simulink model "WSCC_1SM_1GFM_1GFL"  (R2020b)
settings: Solver=VariableStepAuto  StartTime=0.0  StopTime=simlt.T_stop  RelTol=1e-3
undefined symbols (not defined in the file or in its folder): simlt
libraries: powerlib x45, G2ELib_V1 x3, eePowerMeasurement x3
settings Model: Creator=keladaf  LastModifiedBy=keladaf
settings DataIOCC: ReturnWorkspaceOutputs=off
settings DebuggingCC: UnconnectedInputMsg=none  UnconnectedOutputMsg=none  UnconnectedLineMsg=none

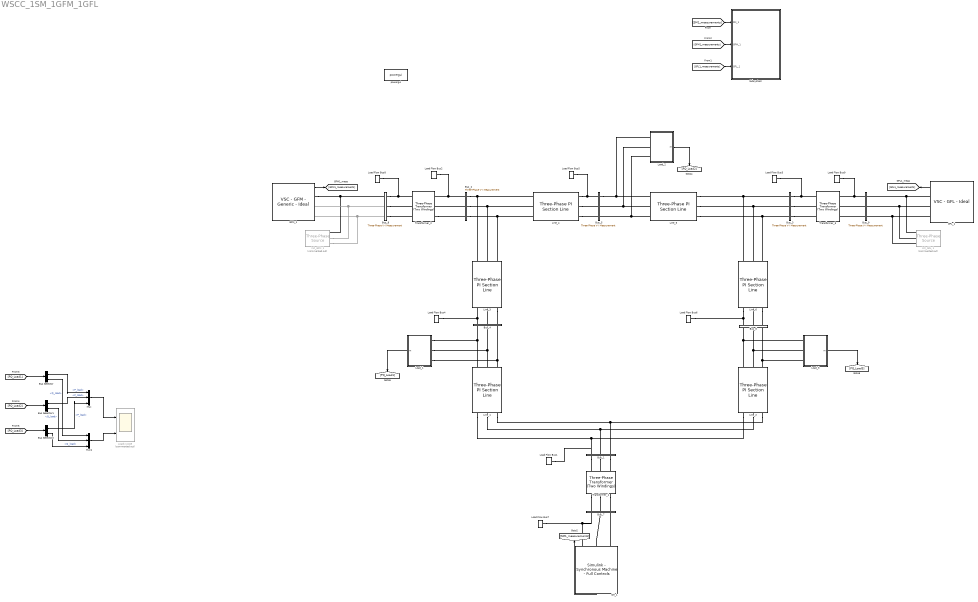
== system WSCC_1SM_1GFM_1GFL ==
  Bus Selector : BusSelector  OutputSignals=P_load,Q_load
  Bus Selector1 : BusSelector  OutputSignals=P_load,Q_load
  Bus Selector2 : BusSelector  OutputSignals=P_load,Q_load
  Bus_1 : powerlib/Measurements/Three-Phase V-I Measurement  VoltageMeasurement=phase-to-ground  SetLabelV=on  LabelV=V_Bus1  Vpu=off  VpuLL=off  CurrentMeasurement=yes  SetLabelI=on  LabelI=I_Bus1  Ipu=off  Pbase=100e6  Vbase=500e3  OutputType=Complex  PhasorSimulation=off  PSBequivalent=0
  Bus_2 : powerlib/Measurements/Three-Phase V-I Measurement  VoltageMeasurement=phase-to-ground  SetLabelV=on  LabelV=V_Bus2  Vpu=off  VpuLL=off  CurrentMeasurement=yes  SetLabelI=on  LabelI=I_Bus2  Ipu=off  Pbase=100e6  Vbase=500e3  OutputType=Complex  PhasorSimulation=off  PSBequivalent=0
  Bus_3 : powerlib/Measurements/Three-Phase V-I Measurement  VoltageMeasurement=phase-to-ground  SetLabelV=on  LabelV=V_Bus3  Vpu=off  VpuLL=off  CurrentMeasurement=yes  SetLabelI=on  LabelI=I_Bus3  Ipu=off  Pbase=100e6  Vbase=500e3  OutputType=Complex  PhasorSimulation=off  PSBequivalent=0
  Bus_4 : powerlib/Measurements/Three-Phase V-I Measurement  VoltageMeasurement=phase-to-ground  SetLabelV=on  LabelV=V_Bus4  Vpu=off  VpuLL=off  CurrentMeasurement=yes  SetLabelI=on  LabelI=I_Bus4  Ipu=off  Pbase=100e6  Vbase=500e3  OutputType=Complex  PhasorSimulation=off  PSBequivalent=0
  Bus_5 : powerlib/Measurements/Three-Phase V-I Measurement  VoltageMeasurement=phase-to-ground  SetLabelV=on  LabelV=V_Bus5  Vpu=off  VpuLL=off  CurrentMeasurement=yes  SetLabelI=on  LabelI=I_Bus5  Ipu=off  Pbase=100e6  Vbase=500e3  OutputType=Complex  PhasorSimulation=off  PSBequivalent=0
  Bus_6 : powerlib/Measurements/Three-Phase V-I Measurement  VoltageMeasurement=phase-to-ground  SetLabelV=on  LabelV=V_Bus6  Vpu=off  VpuLL=off  CurrentMeasurement=yes  SetLabelI=on  LabelI=I_Bus6  Ipu=off  Pbase=100e6  Vbase=500e3  OutputType=Complex  PhasorSimulation=off  PSBequivalent=0
  Bus_7 : powerlib/Measurements/Three-Phase V-I Measurement  VoltageMeasurement=phase-to-ground  SetLabelV=on  LabelV=V_Bus7  Vpu=off  VpuLL=off  CurrentMeasurement=yes  SetLabelI=on  LabelI=I_Bus7  Ipu=off  Pbase=100e6  Vbase=500e3  OutputType=Complex  PhasorSimulation=off  PSBequivalent=0
  Bus_8 : powerlib/Measurements/Three-Phase V-I Measurement  VoltageMeasurement=phase-to-ground  SetLabelV=on  LabelV=V_Bus8  Vpu=off  VpuLL=off  CurrentMeasurement=yes  SetLabelI=on  LabelI=I_Bus8  Ipu=off  Pbase=100e6  Vbase=500e3  OutputType=Complex  PhasorSimulation=off  PSBequivalent=0
  Bus_9 : powerlib/Measurements/Three-Phase V-I Measurement  VoltageMeasurement=phase-to-ground  SetLabelV=on  LabelV=V_Bus9  Vpu=off  VpuLL=off  CurrentMeasurement=yes  SetLabelI=on  LabelI=I_Bus9  Ipu=off  Pbase=100e6  Vbase=500e3  OutputType=Complex  PhasorSimulation=off  PSBequivalent=0
  GFL_1 : G2ELib_V1/DC//AC Converters/Voltage Source Converters (VSC)/Grid-Following VSC (GFL)/VSC - GFL - Ideal  index_c=1  Parameters_fb=60  Parameters_wb=376.9911  GFL_Un=18000  GFL_Un_dc=29393.8769  GFL_Sn=100000000  GFL_Ib=4536.0921  GFL_Ub=14696.9385  GFL_Ub_dc=29393.8769  GFL_Ib_dc=3402.0691  GFL_Pref=1.05  GFL_Qref=0  GFL_V=1.0233  GFL_Theta_Eg0=0.048949  GFL_Vdcref=29393.8769  Delta_Pref_GFL=0.1  Tsw_Pref_GFL=1  Delta_Qref_GFL=0.1  Tsw_Qref_GFL=200  GFL_DC_link_R=500000  GFL_DC_link_C=0.05  GFL_DC_link_Vdc_init=29393.8769  DC_link_Tdc=1e-3  GFL_R1_pu=0.015  GFL_R2_pu=0.0533  GFL_L1_pu=0.1  GFL_L2_pu=0.00061115  GFL_C_pu=0.11  GFL_R1=0.0486  GFL_R2=0.17269  GFL_L1=0.00085944  GFL_L2=5.2524e-06  GFL_C=9.0057e-05  Controllers=PLL  GFL_Control_PLL=1  GFL_Control_VIM=0  GFL_Control_SU_theta=1  GFL_Control_SU_omega=1  GFL_vdc_Kp=-25.92  GFL_vdc_Ki=-777.8349  GFL_KQ=-30  GFL_Inner_current_loop_Kp=0.14415  GFL_Inner_current_loop_Ki=47.7609  GFL_Inner_current_loop_Kffv=1  PLL_Kp=0.31831  PLL_Ki=19.1044  M_pll_0=-0.052344  VIM_wc=18.8496  VIM_wc_ini=0  VIM_Iqd_sat=0.25  VIM_Rr_pu=0.0005  VIM_Lr_pu=0.05  VIM_Lm_pu=0.6  VIM_Rr=0.00162  VIM_Lr=0.00042972  VIM_Lm=0.0051566  VIM_Kp=3.7699  VIM_Kd=0.001  VIM_Nd=100  VIM_H=5.04  VIM_J=0.0070925  VIM_D=0.8  VIM_Inertia_ini=0  VIM_Ke_ini=0  VIM_T_sync=0  VIM_f0=50  VIM_w0=0.83333  GFL_Inner_current_loop_Int_ini_d=0.015391  GFL_Inner_current_loop_Int_ini_q=0.0016885  GFL_Filter_I_ini="[ 737.73244     -4373.1238      3635.3914 ]"  GFL_Filter_V_ini="[ 735.888716     -13377.3055      12641.4168 ]"  GFL_Line_I_ini="[ 227.7291     -4139.7588      3912.0297 ]"  GFL_Is0_dq0="[ 1.0261     0.11257           0 ]"  GFL_Eg0_dq0="[ 1.0233           0           0 ]"  GFL_Ig0_dq0="[ 1.0261           0           0 ]"  GFL_Vm0_dq0="[ 1.0275     0.10429           0 ]"  M_d_0=-0.0013191  M_q_0=-0.0037522  GFL_theta=0.048949
  GFM_1 : G2ELib_V1/DC//AC Converters/Voltage Source Converters (VSC)/Grid-Forming VSC (GFM)/VSC - GFM - Generic - Ideal  index_c=1  Parameters_fb=60  Parameters_wb=376.9911  GFM_Un=18000  GFM_Un_dc=29393.8769  GFM_Sn=100000000  GFM_Ib=4536.0921  GFM_Ub=14696.9385  GFM_Ub_dc=29393.8769  GFM_Ib_dc=3402.0691  GFM_Pref=1.05  GFM_Qref=-0.070519  GFM_Vref=1  GFM_Theta_Eg0=0.039861  GFM_Vdcref=29393.8769  Delta_Pref_GFM=-0.1  Tsw_Pref_GFM=2  Delta_Vref_GFM=-0.01  Tsw_Vref_GFM=300  DC_link_R=500000  DC_link_C=0.05  DC_link_Vdc_init=29393.8769  DC_link_Tdc=0.001  GFM_R1_pu=0.01  GFM_R2_pu=0.0533  GFM_L1_pu=0.1  GFM_L2_pu=0.00061115  GFM_C_pu=0.1  GFM_R1=0.0324  GFM_R2=0.17269  GFM_L1=0.00085944  GFM_L2=5.2524e-06  GFM_C=8.187e-05  Controllers=Droop  Control_PLL=0  Control_VIM=0  Control_MMU_QVDroop=1  Control_MMU_VSM=0  Control_dVOC=0  Control_MMU=1  Control_SU_PfDroop=1  Control_SU_Matching=0  Control_SU_VSM=0  Control_SU_theta=2  Control_SU_omega=2  Control_omega_set=2  Droop_mp=0.005  Droop_nq=0.0001  Droop_wc=33.3333  Droop_Int_ini=0  q_filter_wf=33.3333  q_filter_Int_ini=-0.070519  p_filter_Int_ini=1.05  dVOC_eta=0.005  dVOC_alpha=5000  Matching_K_theta=1.296  VSM_D=200  VSM_J=6  VSM_AVR_Kp=0.05  VSM_AVR_Ki=11.64  VSM_Dq=10000  VSM_K=300  Vdc_loop_Ki=0  Vdc_loop_Kp=259.2  Vdc_loop_Kffi=1  Vdc_loop_Int_ini=29393.8769  Damping_resistor_Enable=0  Damping_resistor_Rv=-0.052947  Damping_resistor_W_RV=75.3982  VI_Enable=0  VI_Rv_pu=0.01  VI_Lv_pu=0.1  TVI_K_RV=0.60041  TVI_Rho_XR=5  TVI_I_thresh_pu=1.2  Inner_voltage_loop_Kp=0.1061  Inner_voltage_loop_Ki=21.2271  Inner_voltage_loop_Kffi=1  Inner_current_loop_Kp=15.9055  Inner_current_loop_Ki=477609.0672  Inner_current_loop_Kffv=1  PLL_Kp=0.4  PLL_Ki=4.69  PLL_Int_ini=0  VIM_wc=0.1*2*pi*50  VIM_wc_ini=0  VIM_Iqd_sat=0.25  VIM_Rr_pu=0.0005  VIM_Lr_pu=0.05  VIM_Lm_pu=0.6  VIM_Rr=0.0048  VIM_Lr=0.0015  VIM_Lm=0.0183  VIM_Kp=3.1416  VIM_Kd=0.001  VIM_Nd=100  VIM_H=0  VIM_J=0.0043  VIM_D=10  VIM_Inertia_ini=0  VIM_Ke_ini=0  VIM_T_sync=0.01  VIM_f0=50.08  VIM_w0=1.0016  SFR_Enable=0  SFR_Rc=0.001  SFR_dP_max=0.3  Inner_voltage_loop_Int_ini_d=0  Inner_voltage_loop_Int_ini_q=-2.7756e-17  Inner_current_loop_Int_ini_d=0.0105  Inner_current_loop_Int_ini_q=0.0017052  Damping_resistor_Int_ini=0  Filter_I_ini="[ 962.67897     -4576.1581      3613.4792 ]"  Filter_V_ini="[ 585.681965     -13010.6526      12424.9706 ]"  Line_I_ini="[ 509.43008     -4365.1885      3855.7584 ]"  Is0_dq0="[ 1.05     0.17052           0 ]"  Eg0_dq0="[ 1           0           0 ]"  Ig0_dq0="[ 1.05    0.070519           0 ]"  Vm0_dq0="[ 0.99345     0.10671           0 ]"  dVOC_ini_theta=0.039861  dVOC_ini_R0=[1,0;0,1]  Matching_Int_ini=0.039861  GFM_theta=0.039861
  Init_GFL_1 : powerlib/Electrical Sources/Three-Phase Source  Commented=on  InternalConnection=Yg  VoltagePhases=off  Voltage=(18000)*1.02306  PhaseAngle=2.7087  Voltage_phases=[25e3 25e3 25e3]/sqrt(3)  PhaseAngles_phases=[0 -120 +120]  Frequency=60  NonIdealSource=off  SpecifyImpedance=off  Resistance=0.8929  Inductance=16.58e-3  ShortCircuitLevel=100e6  BaseVoltage=18000  XRratio=7  BusType=PQ  Pref=105000000  Qref=0  Prefabc=[10e3, 10e3, 10e3]  Qrefabc=[0, 0, 0]  Qmin=-inf  Qmax=inf
  Init_GFM_1 : powerlib/Electrical Sources/Three-Phase Source  Commented=on  InternalConnection=Yg  VoltagePhases=off  Voltage=(18000)*1  PhaseAngle=2.1922  Voltage_phases=[25e3 25e3 25e3]/sqrt(3)  PhaseAngles_phases=[0 -120 +120]  Frequency=60  NonIdealSource=off  SpecifyImpedance=off  Resistance=0.8929  Inductance=16.58e-3  ShortCircuitLevel=100e6  BaseVoltage=18000  XRratio=7  BusType=PV  Pref=105000000  Qref=-7051881.37  Prefabc=[10e3, 10e3, 10e3]  Qrefabc=[0, 0, 0]  Qmin=-inf  Qmax=inf
  Line_1 : powerlib/Elements/Three-Phase PI Section Line  LConnTagsString=a|b|c  RConnTagsString=A|B|C  Length=1  Frequency=60  Resistances=[ 5.29 0.3864 ]  Inductances=[ 0.11927 0.0041264 ]  Capacitances=[ 8.8252e-07 7.751e-09 ]
  Line_2 : powerlib/Elements/Three-Phase PI Section Line  LConnTagsString=a|b|c  RConnTagsString=A|B|C  Length=1  Frequency=60  Resistances=[ 8.993 0.3864 ]  Inductances=[ 0.1291 0.0041264 ]  Capacitances=[ 7.9226e-07 7.751e-09 ]
  Line_3 : powerlib/Elements/Three-Phase PI Section Line  LConnTagsString=a|b|c  RConnTagsString=A|B|C  Length=1  Frequency=60  Resistances=[ 16.928 0.3864 ]  Inductances=[ 0.22592 0.0041264 ]  Capacitances=[ 1.5344e-06 7.751e-09 ]
  Line_4 : powerlib/Elements/Three-Phase PI Section Line  LConnTagsString=a|b|c  RConnTagsString=A|B|C  Length=1  Frequency=60  Resistances=[ 4.4965 0.3864 ]  Inductances=[ 0.10103 0.0041264 ]  Capacitances=[ 7.4714e-07 7.751e-09 ]
  Line_5 : powerlib/Elements/Three-Phase PI Section Line  LConnTagsString=a|b|c  RConnTagsString=A|B|C  Length=1  Frequency=60  Resistances=[ 6.2951 0.3864 ]  Inductances=[ 0.14144 0.0041264 ]  Capacitances=[ 1.048e-06 7.751e-09 ]
  Line_6 : powerlib/Elements/Three-Phase PI Section Line  LConnTagsString=a|b|c  RConnTagsString=A|B|C  Length=1  Frequency=60  Resistances=[ 20.631 0.3864 ]  Inductances=[ 0.23855 0.0041264 ]  Capacitances=[ 1.7951e-06 7.751e-09 ]
  Load Flow Bus1 : powerlib/Measurements/Load Flow Bus  LConnTagsString=a  Phases=single  Connectors=on one side  ID=BUS_1  Vbase=230000  Vref=1  Vangle=0  VLF=1.013  VLFb=1  VLFc=1  angleLF=-3.469  angleLFb=0  angleLFc=0
  Load Flow Bus2 : powerlib/Measurements/Load Flow Bus  LConnTagsString=a  Phases=single  Connectors=on one side  ID=BUS_2  Vbase=230000  Vref=1  Vangle=0  VLF=1.007  VLFb=1  VLFc=1  angleLF=-1.543  angleLFb=0  angleLFc=0
  Load Flow Bus3 : powerlib/Measurements/Load Flow Bus  LConnTagsString=a  Phases=single  Connectors=on one side  ID=BUS_3  Vbase=230000  Vref=1  Vangle=0  VLF=1.025  VLFb=1  VLFc=1  angleLF=-0.6523  angleLFb=0  angleLFc=0
  Load Flow Bus4 : powerlib/Measurements/Load Flow Bus  LConnTagsString=a  Phases=single  Connectors=on one side  ID=BUS_4  Vbase=230000  Vref=1  Vangle=0  VLF=0.9822  VLFb=1  VLFc=1  angleLF=-6.702  angleLFb=0  angleLFc=0
  Load Flow Bus5 : powerlib/Measurements/Load Flow Bus  LConnTagsString=a  Phases=single  Connectors=on one side  ID=BUS_5  Vbase=230000  Vref=1  Vangle=0  VLF=1.001  VLFb=1  VLFc=1  angleLF=-3.486  angleLFb=0  angleLFc=0
  Load Flow Bus6 : powerlib/Measurements/Load Flow Bus  LConnTagsString=a  Phases=single  Connectors=on one side  ID=BUS_6  Vbase=230000  Vref=1  Vangle=0  VLF=1.002  VLFb=1  VLFc=1  angleLF=-5.454  angleLFb=0  angleLFc=0
  Load Flow Bus7 : powerlib/Measurements/Load Flow Bus  LConnTagsString=a  Phases=single  Connectors=on one side  ID=BUS_7  Vbase=18000  Vref=1.025  Vangle=0  VLF=1.025  VLFb=1  VLFc=1  angleLF=0  angleLFb=0  angleLFc=0
  Load Flow Bus8 : powerlib/Measurements/Load Flow Bus  LConnTagsString=a  Phases=single  Connectors=on one side  ID=BUS_8  Vbase=18000  Vref=1  Vangle=0  VLF=1  VLFb=1  VLFc=1  angleLF=2.192  angleLFb=0  angleLFc=0
  Load Flow Bus9 : powerlib/Measurements/Load Flow Bus  LConnTagsString=a  Phases=single  Connectors=on one side  ID=BUS_9  Vbase=18000  Vref=1  Vangle=0  VLF=1.023  VLFb=1  VLFc=1  angleLF=2.709  angleLFb=0  angleLFc=0
  Load_1 : Subsystem
  Load_2 : Subsystem
  Load_3 : Subsystem
  Loads scope : Scope  Commented=on  NumInputPorts=2
  Mux : Mux  Inputs=3
  Mux1 : Mux  Inputs=3
  SM_1 : G2ELib_V1/Synchronous Machine Models/Simulink - Synchronous Machine - Full Controls  index_SM=1  SM_Sn=100000000  SM_Un=18000  Parameters_fb=60  SM_wr=1  SM_Ra=0.003  SM_Ll=0.15  SM_Lad=1.66  SM_Laq=1.61  SM_L1d=0.1713  SM_R1d=0.0284  SM_L1q=0.7252  SM_R1q=0.00619  SM_L2q=0.125  SM_R2q=0.02368  SM_Rfd=0.0006  SM_Lfd=0.165  SM_H=5  SM_K_D=0  SM_Es_base=14696.9385  SM_Is_base=4536.0921  SM_Pt=1.0853  SM_Qt=0.25432  SM_Et=1.025  SM_It=1.0875  SM_Te_0=1.0889  SM_alpha=0  SM_Phi=0  SM_delta0=0.90443  SM_theta_0=-0.66637  SM_ed_0=0.80572  SM_eq_0=0.63359  SM_id_0=0.98571  SM_iq_0=0.45948  SM_efd_0=2.4191  SM_ifd_0=1.4573  SM_Psi_d0=0.63497  SM_Psi_q0=-0.80868  SM_Psi_fd0=1.0233  SM_Psi_1d0=0.78282  SM_Psi_1q0=-0.73976  SM_Psi_2q0=-0.73976  SM_mp=0.5  SM_Tg=0.2  SM_Tr=0.02  SM_Ka=300  SM_Ta=0.001  SM_Ke=1  SM_Te=0.0001  SM_Tb=0  SM_Tc=0  SM_Kf=0.001  SM_Tf=0.1  SM_Efmin=-11.5  SM_Efmax=11.5  SM_Kp=0  SM_T_LP=0.03  SM_K_PSS=2  SM_T_HP=2  SM_T1n=0.05  SM_T1d=0.02  SM_T2n=3  SM_T2d=5.4  SM_VSmax=0.15  SM_VSmin=-0.15  delta_Pref=0.1  T_Pref=200  delta_Vref=0.01  T_Vref=200
      link override Excitation System: v0=[1.025 2.4285]
      link override Synchronous Machine pu Fundamental: BusType=swing  InitialConditions=[0 -37.9762 1.09424 1.09424 1.09424 -13.0731 -133.073 106.927 2.42852]
      link override Synchronous Machine pu Fundamental2: BusType=swing  InitialConditions=[0 -47.6212 0.828791 0.828791 0.828791 -19.253 -139.253 100.747 2.07832]  LoadFlowParameters=[1 0 0 0 0]
      link override Three-Phase Parallel RLC Load: NominalVoltage=(18000)*1.025
  Subsystem : Subsystem
  Transformer_1 : powerlib/Elements/Three-Phase Transformer (Two Windings)  Winding1Connection=Yg  Winding2Connection=Yg  CoreType=Three single-phase transformers  SetSaturation=off  Hysteresis=off  DataFile='hysteresis'  SetInitialFlux=off  Measurements=None  UNITS=pu  NominalPower=[ 100000000 60 ]  Winding1=[ 230000 0 0.0288 ]  Winding2=[ 18000 0 0.0288 ]  Rm=500  Lm=500  L0=0.5  Saturation=[ 0,0 ; 0.0024,1.2 ; 1.0,1.52 ]  InitialFluxes=[ 0.8 , -0.8 , 0.7 ]  BreakLoop=off  DiscreteSolver=Trapezoidal iterative  DataType=off  TransfoNumber=1
  Transformer_2 : powerlib/Elements/Three-Phase Transformer (Two Windings)  Winding1Connection=Yg  Winding2Connection=Yg  CoreType=Three single-phase transformers  SetSaturation=off  Hysteresis=off  DataFile='hysteresis'  SetInitialFlux=off  Measurements=None  UNITS=pu  NominalPower=[ 100000000 60 ]  Winding1=[ 230000 0 0.03125 ]  Winding2=[ 18000 0 0.03125 ]  Rm=500  Lm=500  L0=0.5  Saturation=[ 0,0 ; 0.0024,1.2 ; 1.0,1.52 ]  InitialFluxes=[ 0.8 , -0.8 , 0.7 ]  BreakLoop=off  DiscreteSolver=Trapezoidal iterative  DataType=off  TransfoNumber=1
  Transformer_3 : powerlib/Elements/Three-Phase Transformer (Two Windings)  Winding1Connection=Yg  Winding2Connection=Yg  CoreType=Three single-phase transformers  SetSaturation=off  Hysteresis=off  DataFile='hysteresis'  SetInitialFlux=off  Measurements=None  UNITS=pu  NominalPower=[ 100000000 60 ]  Winding1=[ 230000 0 0.0293 ]  Winding2=[ 18000 0 0.0293 ]  Rm=500  Lm=500  L0=0.5  Saturation=[ 0,0 ; 0.0024,1.2 ; 1.0,1.52 ]  InitialFluxes=[ 0.8 , -0.8 , 0.7 ]  BreakLoop=off  DiscreteSolver=Trapezoidal iterative  DataType=off  TransfoNumber=1
  powergui : powerlib/powergui  Priority=1  SimulationMode=Discrete  SampleTime=simlt.T_step  frequency=60  Iterations=50  frequencyindice=60  Pbase=100e6  ErrMax=0.0001  UnitsV=kV  UnitsW=MW  buscounter=0  FunctionMessages=off  echomessages=off  EnableUseOfTLC=off  CurrentSourceSwitches=off  DisableSnubberDevices=off  DisableRonSwitches=off  DisableVfSwitches=off  DisplayEquations=off  AutomaticDiscreteSolvers=off  SolverType=Tustin/Backward Euler (TBE)  Interpol=off  ExternalGateDelay=off  methode=off  Ts=100  x0status=blocks  SPID=on  SwTol=0  HookPort=off  NonlinearTolerance=1e-4  nMaxIteration=100  ContinueOnMaxIteration=off  RestoreLinks=warning  ResistiveCurrentMeasurement=off  Frange=[0:2:500]  Ylog=off  Xlog=on  ShowGrid=off  save=off  variable=ZData  structure=0  ZoomFFT=off  StartTime=0.0  cycles=1  DisplayStyle=1  fundamental=60  FreqAxis=off  MaxFrequency=1000  frequencyindicesteady=1  RmsSteady=1  display=off
  wires:
  [SM1_measurements] -> Subsystem/1(SM_1)
  Load_1/1(m) -> [PQ_Load1]
  Load_2/1(m) -> [PQ_Load2]
  Load_3/1(m) -> [PQ_Load3]
  [PQ_Load1] -> Bus Selector/1
  [PQ_Load2] -> Bus Selector1/1
  [PQ_Load3] -> Bus Selector2/1
  Bus Selector/1 -> Mux/1  "<P_load>"
  Bus Selector1/1 -> Mux/2  "<P_load>"
  Bus Selector2/1 -> Mux/3  "<P_load>"
  Bus Selector/2 -> Mux1/1  "<Q_load>"
  Bus Selector1/2 -> Mux1/2  "<Q_load>"
  Bus Selector2/2 -> Mux1/3  "<Q_load>"
  Mux/1 -> Loads scope/1
  Mux1/1 -> Loads scope/2
  GFL_1/1 -> [GFL1_measurements]
  GFM_1/1 -> [GFM1_measurements]
  [GFL1_measurements] -> Subsystem/3(GFL_1)
  [GFM1_measurements] -> Subsystem/2(GFM_1)
  SM_1/1 -> [SM1_measurements]
  connections:
  Line_4/RConn1 -- Load Flow Bus5/LConn1 -- Bus_5/LConn1
  Bus_5/RConn1 -- Line_5/LConn1 -- Load_2/LConn1
  Line_4/RConn2 -- Bus_5/LConn2
  Line_5/LConn2 -- Load_2/LConn2 -- Bus_5/RConn2
  Line_4/RConn3 -- Bus_5/LConn3
  Line_5/LConn3 -- Load_2/LConn3 -- Bus_5/RConn3
  Line_3/LConn1 -- Bus_2/RConn1 -- Line_4/LConn1
  Line_3/LConn2 -- Bus_2/RConn2 -- Line_4/LConn2
  Line_3/LConn3 -- Line_4/LConn3 -- Bus_2/RConn3
  Bus_2/LConn1 -- Load Flow Bus2/LConn1 -- Transformer_2/LConn1
  Bus_2/LConn2 -- Transformer_2/LConn2
  Bus_8/RConn1 -- Load Flow Bus8/LConn1 -- Transformer_2/RConn1
  Bus_8/RConn2 -- Transformer_2/RConn2
  Bus_8/RConn3 -- Transformer_2/RConn3
  Bus_3/RConn2 -- Transformer_3/LConn2
  Bus_3/RConn3 -- Transformer_3/LConn3
  Line_6/LConn1 -- Bus_3/LConn1 -- Line_5/RConn1
  Line_6/LConn2 -- Bus_3/LConn2 -- Line_5/RConn2
  Line_6/LConn3 -- Bus_3/LConn3 -- Line_5/RConn3
  Bus_9/LConn1 -- Load Flow Bus9/LConn1 -- Transformer_3/RConn1
  Bus_9/LConn2 -- Transformer_3/RConn2
  Bus_9/LConn3 -- Transformer_3/RConn3
  Bus_4/LConn1 -- Load Flow Bus4/LConn1 -- Line_3/RConn1
  Line_3/RConn2 -- Bus_4/LConn2
  Line_3/RConn3 -- Bus_4/LConn3
  Line_1/LConn1 -- Bus_4/RConn1 -- Load_1/LConn1
  Line_1/LConn2 -- Load_1/LConn2 -- Bus_4/RConn2
  Line_1/LConn3 -- Load_1/LConn3 -- Bus_4/RConn3
  Line_6/RConn2 -- Bus_6/LConn2
  Line_6/RConn1 -- Load Flow Bus6/LConn1 -- Bus_6/LConn1
  Line_6/RConn3 -- Bus_6/LConn3
  Line_2/LConn3 -- Load_3/LConn3 -- Bus_6/RConn3
  Line_2/LConn2 -- Load_3/LConn2 -- Bus_6/RConn2
  Line_2/LConn1 -- Load_3/LConn1 -- Bus_6/RConn1
  Bus_1/RConn2 -- Transformer_1/LConn2
  Bus_1/RConn3 -- Transformer_1/LConn3
  Line_1/RConn1 -- Load Flow Bus1/LConn1 -- Bus_1/LConn1 -- Line_2/RConn1
  Line_1/RConn2 -- Bus_1/LConn2 -- Line_2/RConn2
  Line_1/RConn3 -- Bus_1/LConn3 -- Line_2/RConn3
  Transformer_1/RConn1 -- Bus_7/LConn1
  Transformer_1/RConn2 -- Bus_7/LConn2
  Transformer_1/RConn3 -- Bus_7/LConn3
  SM_1/LConn1 -- Bus_7/RConn1 -- Load Flow Bus7/LConn1
  GFL_1/RConn1 -- Init_GFL_1/RConn1 -- Bus_9/RConn1
  GFL_1/RConn2 -- Init_GFL_1/RConn2 -- Bus_9/RConn2
  GFL_1/RConn3 -- Init_GFL_1/RConn3 -- Bus_9/RConn3
  Init_GFM_1/RConn3 -- Bus_8/LConn3 -- GFM_1/RConn3
  GFM_1/RConn1 -- Bus_8/LConn1 -- Init_GFM_1/RConn1
  Init_GFM_1/RConn2 -- Bus_8/LConn2 -- GFM_1/RConn2
  SM_1/LConn3 -- Bus_7/RConn3
  SM_1/LConn2 -- Bus_7/RConn2
  Bus_1/RConn1 -- Transformer_1/LConn1
  Transformer_2/LConn3 -- Bus_2/LConn3
  Bus_3/RConn1 -- Load Flow Bus3/LConn1 -- Transformer_3/LConn1

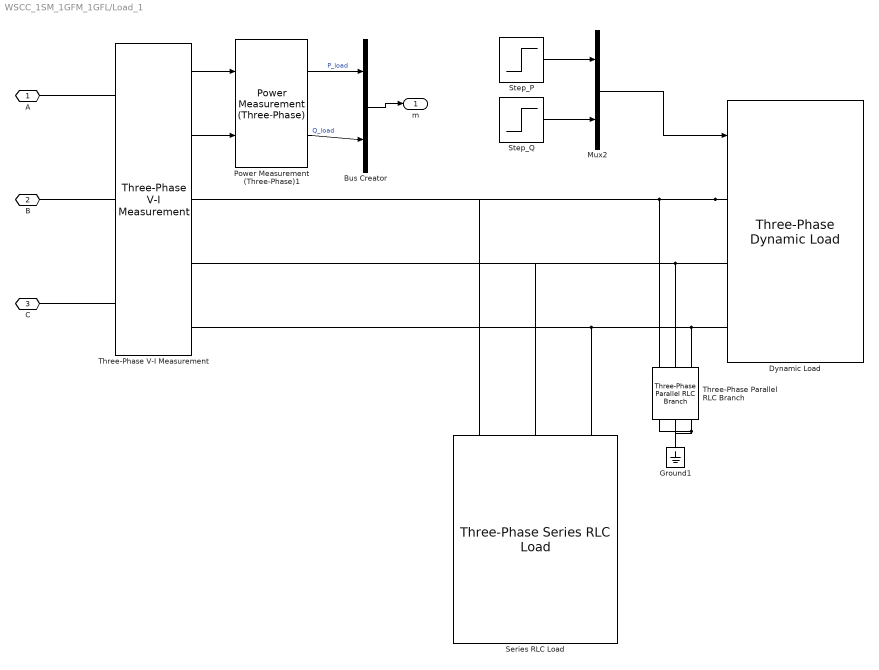
== system WSCC_1SM_1GFM_1GFL/Load_1 ==
  Bus Creator : BusCreator  Inputs=2
  Dynamic Load : powerlib/Elements/Three-Phase Dynamic Load  NominalVoltage=[ 230000 60 ]  ActiveReactivePowers=[0 0]  PositiveSequence=[0.982229 -6.70204]  ExternalControl=on  NpNq=[1.3 2]  TimeConstants="[0  0  0  0]"  MinimumVoltage=0.7  Tfilter=1e-4  LoadFlowParameters=[4,0,0,0,0]
      settings: SourceProductBaseCode=PS
  Ground1 : powerlib/Elements/Ground  LConnTagsString=a
  Mux2 : Mux  Inputs=2
  Power Measurement (Three-Phase)1 : eePowerMeasurement/Power Measurement (Three-Phase)  LabelModeActiveChoice=Continuous  F=Parameters.fb  K=1  Seq=Positive  Ts=0
      settings: SourceProductBaseCode=PS
  Series RLC Load : powerlib/Elements/Three-Phase Series RLC Load  LConnTagsString=A|B|C  Configuration=Y (grounded)  NominalVoltage=(230000)*0.982229  Vabc=[1e3 1e3 1e3]  Vabcp=[1e3 1e3 1e3]  NominalFrequency=60  UnbalancedPower=off  ActivePower=125000000  InductivePower=50000000  CapacitivePower=0  Pabc=[10e3 9e3 11e3]  QLabc=[100 90 110]  QCabc=[100 90 110]  Pabcp=[10e3 9e3 11e3]  QLabcp=[100 90 110]  QCabcp=[100 90 110]  Measurements=None  LoadType=constant PQ
  Step_P : Step  SampleTime=0  mask{StepV=15750000, StepT=250}
      mask prompts: StepV "Step Value (W or VAr)"; StepT "Step time (s)"
      mask DialogControl DescTextVar Prompt: A step change in active or reactive power
  Step_Q : Step  SampleTime=0  mask{StepV=1150000, StepT=500}
      mask prompts: StepV "Step Value (W or VAr)"; StepT "Step time (s)"
      mask DialogControl DescTextVar Prompt: A step change in active or reactive power
  Three-Phase Parallel RLC Branch : powerlib/Elements/Three-Phase Parallel RLC Branch  LConnTagsString=A|B|C  RConnTagsString=A|B|C  BranchType=R  Resistance=1e6  Inductance=1e-3  Capacitance=1e-6  Measurements=None
      settings: SourceProductBaseCode=PS
  Three-Phase V-I Measurement : powerlib/Measurements/Three-Phase V-I Measurement  VoltageMeasurement=phase-to-ground  SetLabelV=off  LabelV=Vabc  Vpu=off  VpuLL=off  CurrentMeasurement=yes  SetLabelI=off  LabelI=Iabc  Ipu=off  Pbase=100e6  Vbase=500e3  OutputType=Complex  PhasorSimulation=off  PSBequivalent=0
  A : PMIOPort  Side=Left
  B : PMIOPort  Port=2  Side=Left
  C : PMIOPort  Port=3  Side=Left
  m : Outport
  wires:
  Three-Phase V-I Measurement/2 -> Power Measurement (Three-Phase)1/2
  Mux2/1 -> Dynamic Load/1
  Step_Q/1 -> Mux2/2
  Power Measurement (Three-Phase)1/2 -> Bus Creator/2  "Q_load"
  Three-Phase V-I Measurement/1 -> Power Measurement (Three-Phase)1/1
  Power Measurement (Three-Phase)1/1 -> Bus Creator/1  "P_load"
  Bus Creator/1 -> m/1
  Step_P/1 -> Mux2/1
  connections:
  Three-Phase Parallel RLC Branch/LConn2 -- Three-Phase V-I Measurement/RConn2 -- Series RLC Load/LConn2 -- Dynamic Load/LConn2
  Dynamic Load/LConn1 -- Three-Phase Parallel RLC Branch/LConn1 -- Three-Phase V-I Measurement/RConn1 -- Series RLC Load/LConn1
  Three-Phase Parallel RLC Branch/RConn3 -- Three-Phase Parallel RLC Branch/RConn2 -- Ground1/LConn1 -- Three-Phase Parallel RLC Branch/RConn1
  Three-Phase V-I Measurement/RConn3 -- Series RLC Load/LConn3 -- Three-Phase Parallel RLC Branch/LConn3 -- Dynamic Load/LConn3
  B/RConn1 -- Three-Phase V-I Measurement/LConn2
  A/RConn1 -- Three-Phase V-I Measurement/LConn1
  C/RConn1 -- Three-Phase V-I Measurement/LConn3

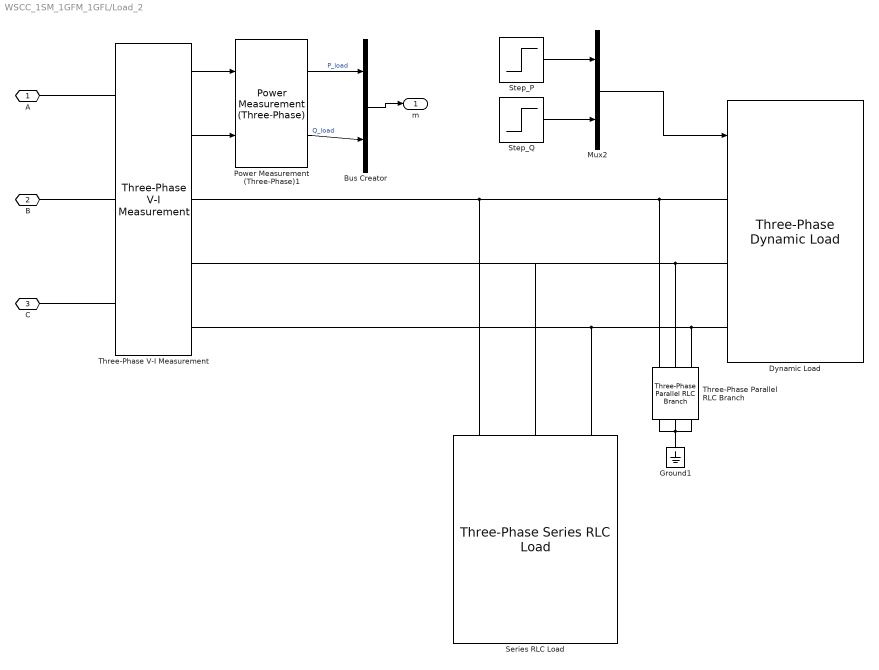
== system WSCC_1SM_1GFM_1GFL/Load_2 ==
  Bus Creator : BusCreator  Inputs=2
  Dynamic Load : powerlib/Elements/Three-Phase Dynamic Load  NominalVoltage=[ 230000 60 ]  ActiveReactivePowers=[0 0]  PositiveSequence=[1.00126 -3.48592]  ExternalControl=on  NpNq=[1.3 2]  TimeConstants="[0  0  0  0]"  MinimumVoltage=0.7  Tfilter=1e-4  LoadFlowParameters=[4,0,0,0,0]
      settings: SourceProductBaseCode=PS
  Ground1 : powerlib/Elements/Ground  LConnTagsString=a
  Mux2 : Mux  Inputs=2
  Power Measurement (Three-Phase)1 : eePowerMeasurement/Power Measurement (Three-Phase)  LabelModeActiveChoice=Continuous  F=Parameters.fb  K=1  Seq=Positive  Ts=0
      settings: SourceProductBaseCode=PS
  Series RLC Load : powerlib/Elements/Three-Phase Series RLC Load  LConnTagsString=A|B|C  Configuration=Y (grounded)  NominalVoltage=(230000)*1.00126  Vabc=[1e3 1e3 1e3]  Vabcp=[1e3 1e3 1e3]  NominalFrequency=60  UnbalancedPower=off  ActivePower=100000000  InductivePower=35000000  CapacitivePower=0  Pabc=[10e3 9e3 11e3]  QLabc=[100 90 110]  QCabc=[100 90 110]  Pabcp=[10e3 9e3 11e3]  QLabcp=[100 90 110]  QCabcp=[100 90 110]  Measurements=None  LoadType=constant PQ
  Step_P : Step  SampleTime=0  mask{StepV=15750000, StepT=250}
      mask prompts: StepV "Step Value (MW or MVAr)"; StepT "Step time (s)"
      mask DialogControl DescTextVar Prompt: A step change in active or reactive power
  Step_Q : Step  SampleTime=0  mask{StepV=1150000, StepT=500}
      mask prompts: StepV "Step Value (W or VAr)"; StepT "Step time (s)"
      mask DialogControl DescTextVar Prompt: A step change in active or reactive power
  Three-Phase Parallel RLC Branch : powerlib/Elements/Three-Phase Parallel RLC Branch  LConnTagsString=A|B|C  RConnTagsString=A|B|C  BranchType=R  Resistance=1e6  Inductance=1e-3  Capacitance=1e-6  Measurements=None
      settings: SourceProductBaseCode=PS
  Three-Phase V-I Measurement : powerlib/Measurements/Three-Phase V-I Measurement  VoltageMeasurement=phase-to-ground  SetLabelV=off  LabelV=Vabc  Vpu=off  VpuLL=off  CurrentMeasurement=yes  SetLabelI=off  LabelI=Iabc  Ipu=off  Pbase=100e6  Vbase=500e3  OutputType=Complex  PhasorSimulation=off  PSBequivalent=0
  A : PMIOPort  Side=Left
  B : PMIOPort  Port=2  Side=Left
  C : PMIOPort  Port=3  Side=Left
  m : Outport
  wires:
  Bus Creator/1 -> m/1
  Step_P/1 -> Mux2/1
  Power Measurement (Three-Phase)1/1 -> Bus Creator/1  "P_load"
  Three-Phase V-I Measurement/1 -> Power Measurement (Three-Phase)1/1
  Power Measurement (Three-Phase)1/2 -> Bus Creator/2  "Q_load"
  Step_Q/1 -> Mux2/2
  Mux2/1 -> Dynamic Load/1
  Three-Phase V-I Measurement/2 -> Power Measurement (Three-Phase)1/2
  connections:
  C/RConn1 -- Three-Phase V-I Measurement/LConn3
  A/RConn1 -- Three-Phase V-I Measurement/LConn1
  B/RConn1 -- Three-Phase V-I Measurement/LConn2
  Series RLC Load/LConn3 -- Three-Phase V-I Measurement/RConn3 -- Dynamic Load/LConn3 -- Three-Phase Parallel RLC Branch/LConn3
  Three-Phase Parallel RLC Branch/RConn2 -- Three-Phase Parallel RLC Branch/RConn3 -- Three-Phase Parallel RLC Branch/RConn1 -- Ground1/LConn1
  Series RLC Load/LConn1 -- Three-Phase V-I Measurement/RConn1 -- Dynamic Load/LConn1 -- Three-Phase Parallel RLC Branch/LConn1
  Three-Phase V-I Measurement/RConn2 -- Series RLC Load/LConn2 -- Three-Phase Parallel RLC Branch/LConn2 -- Dynamic Load/LConn2

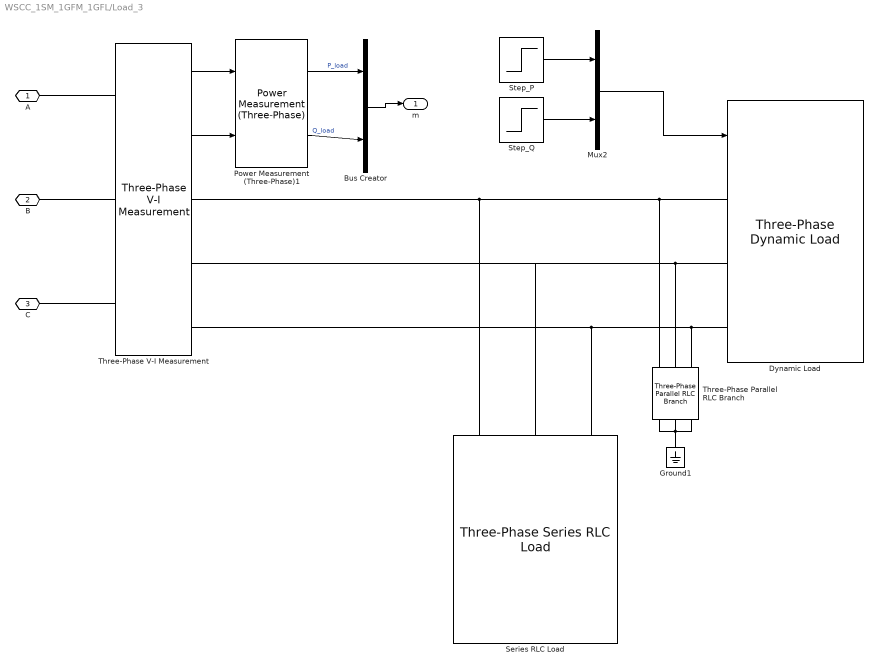
== system WSCC_1SM_1GFM_1GFL/Load_3 ==
  Bus Creator : BusCreator  Inputs=2
  Dynamic Load : powerlib/Elements/Three-Phase Dynamic Load  NominalVoltage=[ 230000 60 ]  ActiveReactivePowers=[0 0]  PositiveSequence=[1.0018 -5.45382]  ExternalControl=on  NpNq=[1.3 2]  TimeConstants="[0  0  0  0]"  MinimumVoltage=0.7  Tfilter=1e-4  LoadFlowParameters=[4,0,0,0,0]
      settings: SourceProductBaseCode=PS
  Ground1 : powerlib/Elements/Ground  LConnTagsString=a
  Mux2 : Mux  Inputs=2
  Power Measurement (Three-Phase)1 : eePowerMeasurement/Power Measurement (Three-Phase)  LabelModeActiveChoice=Continuous  F=Parameters.fb  K=1  Seq=Positive  Ts=0
      settings: SourceProductBaseCode=PS
  Series RLC Load : powerlib/Elements/Three-Phase Series RLC Load  LConnTagsString=A|B|C  Configuration=Y (grounded)  NominalVoltage=(230000)*1.0018  Vabc=[1e3 1e3 1e3]  Vabcp=[1e3 1e3 1e3]  NominalFrequency=60  UnbalancedPower=off  ActivePower=90000000  InductivePower=30000000  CapacitivePower=0  Pabc=[10e3 9e3 11e3]  QLabc=[100 90 110]  QCabc=[100 90 110]  Pabcp=[10e3 9e3 11e3]  QLabcp=[100 90 110]  QCabcp=[100 90 110]  Measurements=None  LoadType=constant PQ
  Step_P : Step  SampleTime=0  mask{StepV=15750000, StepT=250}
      mask prompts: StepV "Step Value (MW or MVAr)"; StepT "Step time (s)"
      mask DialogControl DescTextVar Prompt: A step change in active or reactive power
  Step_Q : Step  SampleTime=0  mask{StepV=1150000, StepT=500}
      mask prompts: StepV "Step Value (W or VAr)"; StepT "Step time (s)"
      mask DialogControl DescTextVar Prompt: A step change in active or reactive power
  Three-Phase Parallel RLC Branch : powerlib/Elements/Three-Phase Parallel RLC Branch  LConnTagsString=A|B|C  RConnTagsString=A|B|C  BranchType=R  Resistance=1e6  Inductance=1e-3  Capacitance=1e-6  Measurements=None
      settings: SourceProductBaseCode=PS
  Three-Phase V-I Measurement : powerlib/Measurements/Three-Phase V-I Measurement  VoltageMeasurement=phase-to-ground  SetLabelV=off  LabelV=Vabc  Vpu=off  VpuLL=off  CurrentMeasurement=yes  SetLabelI=off  LabelI=Iabc  Ipu=off  Pbase=100e6  Vbase=500e3  OutputType=Complex  PhasorSimulation=off  PSBequivalent=0
  A : PMIOPort  Side=Left
  B : PMIOPort  Port=2  Side=Left
  C : PMIOPort  Port=3  Side=Left
  m : Outport
  wires:
  Bus Creator/1 -> m/1
  Step_P/1 -> Mux2/1
  Power Measurement (Three-Phase)1/1 -> Bus Creator/1  "P_load"
  Three-Phase V-I Measurement/1 -> Power Measurement (Three-Phase)1/1
  Power Measurement (Three-Phase)1/2 -> Bus Creator/2  "Q_load"
  Step_Q/1 -> Mux2/2
  Mux2/1 -> Dynamic Load/1
  Three-Phase V-I Measurement/2 -> Power Measurement (Three-Phase)1/2
  connections:
  C/RConn1 -- Three-Phase V-I Measurement/LConn3
  A/RConn1 -- Three-Phase V-I Measurement/LConn1
  B/RConn1 -- Three-Phase V-I Measurement/LConn2
  Series RLC Load/LConn3 -- Three-Phase V-I Measurement/RConn3 -- Dynamic Load/LConn3 -- Three-Phase Parallel RLC Branch/LConn3
  Three-Phase Parallel RLC Branch/RConn2 -- Three-Phase Parallel RLC Branch/RConn3 -- Three-Phase Parallel RLC Branch/RConn1 -- Ground1/LConn1
  Series RLC Load/LConn1 -- Three-Phase V-I Measurement/RConn1 -- Dynamic Load/LConn1 -- Three-Phase Parallel RLC Branch/LConn1
  Three-Phase V-I Measurement/RConn2 -- Series RLC Load/LConn2 -- Three-Phase Parallel RLC Branch/LConn2 -- Dynamic Load/LConn2

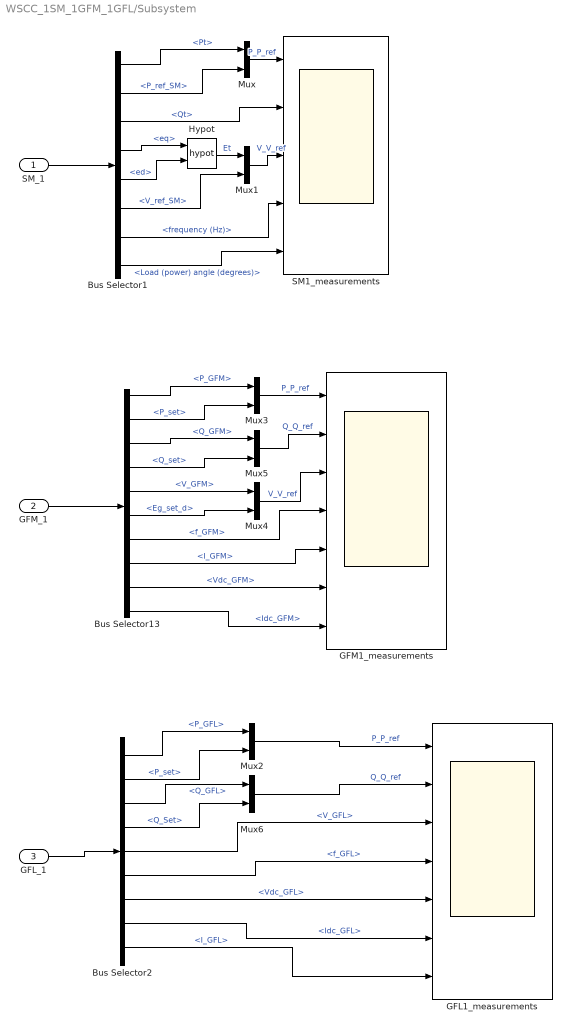
== system WSCC_1SM_1GFM_1GFL/Subsystem ==
  SM_1 : Inport
  GFM_1 : Inport  Port=2
  GFL_1 : Inport  Port=3
  Bus Selector1 : BusSelector  OutputSignals=Terminal Powers (pu).Pt,References (P;V).P_ref_SM,Terminal Powers (pu).Qt,Terminal voltage dq-comp and field voltage (pu).eq,Terminal voltage dq-comp and field voltage (pu).ed,References (P;V).V_ref_SM,frequency (Hz),Load (power) angle (degrees)
  Bus Selector13 : BusSelector  OutputSignals=P_GFM,Setpoints.P_set,Q_GFM,Setpoints.Q_set,V_GFM,Setpoints.Eg_set_d,f_GFM,I_GFM,Vdc_GFM,Idc_GFM
  Bus Selector2 : BusSelector  OutputSignals=P_GFL,Setpoints.P_set,Q_GFL,Setpoints.Q_Set,V_GFL,f_GFL,Vdc_GFL,Idc_GFL,I_GFL
  GFL1_measurements : Scope  NumInputPorts=7
  GFM1_measurements : Scope  NumInputPorts=7
  Hypot : Math  Operator=hypot  SaturateOnIntegerOverflow=on
  Mux{,1..6} (7 alike) : Mux  Inputs=2
  SM1_measurements : Scope  NumInputPorts=5
  wires:
  SM_1/1 -> Bus Selector1/1
  Mux/1 -> SM1_measurements/1  "P_P_ref"
  Bus Selector1/1 -> Mux/1  "<Pt>"
  Bus Selector1/2 -> Mux/2  "<P_ref_SM>"
  Bus Selector1/3 -> SM1_measurements/2  "<Qt>"
  Bus Selector1/4 -> Hypot/1  "<eq>"
  Bus Selector1/5 -> Hypot/2  "<ed>"
  Hypot/1 -> Mux1/1  "Et"
  Bus Selector1/6 -> Mux1/2  "<V_ref_SM>"
  Mux1/1 -> SM1_measurements/3  "V_V_ref"
  Bus Selector1/7 -> SM1_measurements/4  "<frequency (Hz)>"
  Bus Selector1/8 -> SM1_measurements/5  "<Load (power) angle (degrees)>"
  Bus Selector2/7 -> GFL1_measurements/5  "<Vdc_GFL>"
  Bus Selector2/9 -> GFL1_measurements/7  "<I_GFL>"
  Bus Selector2/4 -> Mux6/2  "<Q_Set>"
  Bus Selector2/5 -> GFL1_measurements/3  "<V_GFL>"
  Mux2/1 -> GFL1_measurements/1  "P_P_ref"
  Bus Selector2/6 -> GFL1_measurements/4  "<f_GFL>"
  Bus Selector2/2 -> Mux2/2  "<P_set>"
  Bus Selector2/1 -> Mux2/1  "<P_GFL>"
  Bus Selector2/3 -> Mux6/1  "<Q_GFL>"
  Mux6/1 -> GFL1_measurements/2  "Q_Q_ref"
  Bus Selector2/8 -> GFL1_measurements/6  "<Idc_GFL>"
  GFL_1/1 -> Bus Selector2/1
  Bus Selector13/3 -> Mux5/1  "<Q_GFM>"
  Mux5/1 -> GFM1_measurements/2  "Q_Q_ref"
  GFM_1/1 -> Bus Selector13/1
  Mux3/1 -> GFM1_measurements/1  "P_P_ref"
  Bus Selector13/7 -> GFM1_measurements/4  "<f_GFM>"
  Bus Selector13/5 -> Mux4/1  "<V_GFM>"
  Bus Selector13/1 -> Mux3/1  "<P_GFM>"
  Bus Selector13/4 -> Mux5/2  "<Q_set>"
  Mux4/1 -> GFM1_measurements/3  "V_V_ref"
  Bus Selector13/9 -> GFM1_measurements/6  "<Vdc_GFM>"
  Bus Selector13/10 -> GFM1_measurements/7  "<Idc_GFM>"
  Bus Selector13/8 -> GFM1_measurements/5  "<I_GFM>"
  Bus Selector13/6 -> Mux4/2  "<Eg_set_d>"
  Bus Selector13/2 -> Mux3/2  "<P_set>"
